simulink model "PubIfDecisionTOS_MDL"  (R2020b)
settings: configuration reference "DspaceConfig" (kept outside this file)
PostLoadFcn:
  | if any(exist('dsrtsu_mdlpostloadfcn', 'file') ~= 0), dsrtsu_mdlpostloadfcn('Execute', bdroot); end
InitFcn:
  | , if any(exist('dsmpb_private', 'file') ~= 0), dsmpb_private('dsmpb_mdlclblib', 'Init', bdroot); end,
undefined symbols (not defined in the file or in its folder): C_TOS_ACCEgoRAxletoFbumplength_m, C_TOS_ACCTargetFront_Flag, C_TOS_AEBJAPedObjDxThre_Val, C_TOS_AEBJAPedObjDyThre_Val, C_TOS_AEBJATargetSize_Val, C_TOS_AEBJAVehObjDxThre_Val, C_TOS_AEBJAVehObjDyThre_Val, C_TOS_AEBJuncPedTargetSize_Val, C_TOS_AEBLatObjDxThre_Val, C_TOS_AEBLatPedDyThre_Val, C_TOS_AEBLatTargetSize_Val, C_TOS_AEBLongTargetInEgoFront_Flag, C_TOS_axAbsGround_Parameter, C_TOS_CameraConfirmedFlag, C_TOS_CNsubjWidth, C_TOS_CurrentLaneCoreMinWidth_Val, C_TOS_CutInProb_Val_Zero, C_TOS_CutOutProb_Val_Zero, C_TOS_D2R_Val, C_TOS_DefaultValueObjectToCenterLine_dy, C_TOS_EgoCarWidth_Val, C_TOS_EgoDxRefPoint_m, C_TOS_EgoRAxletoFbumplength_m, C_TOS_HalfWidthVehicle_Con, C_TOS_HWA_CurrentLaneFlag, C_TOS_HWA_LeftLaneFlag, C_TOS_HWA_MovingDir_Vaild, C_TOS_HWA_MovState_Vaild, C_TOS_HWA_RightLaneFlag, C_TOS_LaneLineCourseErrorFront, C_TOS_LaneLineCourseErrorRear, C_TOS_MotorbikeDefaultWidth_m, C_TOS_NumberOfEffectiveTargets, C_TOS_Obj_Age_Val, C_TOS_Objdx_Constraint_Val, C_TOS_ObjectDefaultWidth_m, C_TOS_ObjInCurrentLane_Val, C_TOS_ObjInCurrentLaneValid, C_TOS_ObjInLeftLaneValid, C_TOS_ObjInRightLaneValid, C_TOS_ObjNotInCurrentLane_Val, C_TOS_ObjNotREElementType, C_TOS_ObjPredictDis_dy_ConstantVal_Zeros, C_TOS_ObjToCenterLine_ConstantVal_Zeros, C_TOS_OFMObjIDInvilad_Val, C_TOS_PIL_LatDisCons_Val_zero, C_TOS_PIL_ObjectCutInFlag_b, C_TOS_PIL_ObjectCutOutFlag_b, C_TOS_PIL_ObjLaneProb_al_Val, C_TOS_PP_ObjFusType_FC_Confirm_b, C_TOS_PP_ObjFusType_FC_FR_Confirm_b, C_TOS_PP_ObjFusType_FR_Confirm_b, C_TOS_RE_80BoolDefault_Val, C_TOS_RE_80Single181Default_Val, C_TOS_RE_80Single255Default_Val, C_TOS_RE_80Uint8Default_Val, C_TOS_RE_D2R, C_TOS_RE_D_180_Val, C_TOS_RE_InvalidObjectID_Val, C_TOS_RE_InvalidTargetChainDir_Val ... (+142)
libraries: simulink x1650, TOS_LIB x361, canfdmsglib x14
(part 14 of 69)

== system PubIfDecisionTOS_MDL/TOS_20201112/TOS_2012080320/TOS/P0_Trajectory_V1.0/CordinatConvert/CordinatConvert1 ==
  note: 0x0: not standstill
  EgoVeh_OffsetX : Inport
  EgoVeh_OffsetY : Inport  Port=2
  EgoVeh_OffsetAngle : Inport  Port=3
  VxvRef_ms : Inport  Port=4
  VehStandstill : Inport  Port=5
  P0_dx_TrackRecord_K1 : Inport  Port=6
  P0_dy_TrackRecord_K1 : Inport  Port=7
  P0_Counter_TrackRecord_K1 : Inport  Port=8
  P0_ID_TrackRecord_K1 : Inport  Port=9
  Bus Creator : BusCreator  Inputs=9
  Bus Selector : BusSelector  OutputSignals=VehStandstill
  Bus Selector1 : BusSelector  OutputSignals=EgoVeh_OffsetX,EgoVeh_OffsetY,EgoVeh_OffsetAngle,P0_dx_TrackRecord_K1,P0_dy_TrackRecord_K1,P0_Counter_TrackRecord_K1,P0_ID_TrackRecord_K1
  Bus Selector2 : BusSelector  OutputSignals=VxvRef_ms
  Compare To Constant1 : simulink/Logic and Bit Operations/Compare To Constant  relop===  const=boolean(0)  OutDataTypeStr=boolean
      settings: AttributesFormatString=boolean(0)
  Compare To Constant2 : simulink/Logic and Bit Operations/Compare To Constant  relop=<  const=single(0.4166)  OutDataTypeStr=boolean
      settings: AttributesFormatString=single(0.4166)
  CordinatConvert : Subsystem  TreatAsAtomicUnit=on
  CordinatConvertDefault : Subsystem  TreatAsAtomicUnit=on
  If : If  IfExpression=u1 == 0
  Logical Operator2 : Logic  Operator=OR  AllPortsSameDT=off  OutDataTypeStr=boolean
  Merge{1..4} (4 alike) : Merge
  P0_dx_TrackRecord_CordinatConvert_K1 : Outport
  P0_dy_TrackRecord_CordinatConvert_K1 : Outport  Port=2
  P0_Counter_TrackRecord_CordinatConvert_K1 : Outport  Port=3
  P0_ID_TrackRecord_CordinatConvert_K1 : Outport  Port=4
  wires:
  Compare To Constant1/1 -> Logical Operator2/1
  Logical Operator2/1 -> If/1
  Compare To Constant2/1 -> Logical Operator2/2
  Bus Selector2/1 -> Compare To Constant2/1  "<VxvRef_ms>"
  VxvRef_ms/1 -> Bus Creator/4  "VxvRef_ms"
  CordinatConvert/4(P0_ID_TrackRecord_CordinatConvert_K1) -> Merge4/1
  CordinatConvertDefault/4(P0_ID_TrackRecord_CordinatConvert_K1) -> Merge4/2
  Merge4/1 -> P0_ID_TrackRecord_CordinatConvert_K1/1
  Bus Selector1/7 -> CordinatConvert/7(P0_ID_TrackRecord_K1)  "<P0_ID_TrackRecord_K1>"
  P0_ID_TrackRecord_K1/1 -> Bus Creator/9  "P0_ID_TrackRecord_K1"
  If/2 -> CordinatConvertDefault/Action
  If/1 -> CordinatConvert/Action
  EgoVeh_OffsetX/1 -> Bus Creator/1  "EgoVeh_OffsetX"
  EgoVeh_OffsetY/1 -> Bus Creator/2  "EgoVeh_OffsetY"
  EgoVeh_OffsetAngle/1 -> Bus Creator/3  "EgoVeh_OffsetAngle"
  VehStandstill/1 -> Bus Creator/5  "VehStandstill"
  P0_dx_TrackRecord_K1/1 -> Bus Creator/6  "P0_dx_TrackRecord_K1"
  P0_dy_TrackRecord_K1/1 -> Bus Creator/7  "P0_dy_TrackRecord_K1"
  P0_Counter_TrackRecord_K1/1 -> Bus Creator/8  "P0_Counter_TrackRecord_K1"
  Bus Creator/1 -> [CordinatConvert_Sig], Bus Selector/1, Bus Selector2/1
  Bus Selector/1 -> Compare To Constant1/1  "<VehStandstill>"
  [CordinatConvert_Sig] -> Bus Selector1/1
  CordinatConvertDefault/3(P0_Counter_TrackRecord_CordinatConvert_K1) -> Merge1/2
  CordinatConvertDefault/2(P0_dy_TrackRecord_CordinatConvert_K1) -> Merge3/2
  CordinatConvertDefault/1(P0_dx_TrackRecord_CordinatConvert_K1) -> Merge2/2
  Bus Selector1/1 -> CordinatConvert/1(EgoVeh_OffsetX)  "<EgoVeh_OffsetX>"
  Bus Selector1/2 -> CordinatConvert/2(EgoVeh_OffsetY)  "<EgoVeh_OffsetY>"
  Bus Selector1/3 -> CordinatConvert/3(EgoVeh_OffsetAngle)  "<EgoVeh_OffsetAngle>"
  Bus Selector1/4 -> CordinatConvert/4(P0_dx_TrackRecord_K1)  "<P0_dx_TrackRecord_K1>"
  Bus Selector1/5 -> CordinatConvert/5(P0_dy_TrackRecord_K1)  "<P0_dy_TrackRecord_K1>"
  Bus Selector1/6 -> CordinatConvert/6(P0_Counter_TrackRecord)  "<P0_Counter_TrackRecord_K1>"
  CordinatConvert/1(P0_dx_TrackRecord_CordinatConvert_K1) -> Merge2/1
  CordinatConvert/2(P0_dy_TrackRecord_CordinatConvert_K1) -> Merge3/1
  CordinatConvert/3(P0_Counter_TrackRecord_CordinatConvert_K1) -> Merge1/1
  Merge2/1 -> P0_dx_TrackRecord_CordinatConvert_K1/1
  Merge3/1 -> P0_dy_TrackRecord_CordinatConvert_K1/1
  Merge1/1 -> P0_Counter_TrackRecord_CordinatConvert_K1/1

== system PubIfDecisionTOS_MDL/TOS_20201112/TOS_2012080320/TOS/P0_Trajectory_V1.0/CordinatConvert/EgoVehicleOffset ==
  note: rcs-reference coordinate system
  PsiDtOpt : Inport
  VxvRef_ms : Inport  Port=2
  Compare To Zero : simulink/Logic and Bit Operations/Compare To Zero  relop===  OutDataTypeStr=boolean
  Constant3 : Constant  Value=0  OutDataTypeStr=single
  Constant4 : Constant  Value=P_TOS_SysCycTime_Val
  Constant5 : Constant  OutDataTypeStr=single
  Constant6 : Constant  Value=P_TOS_SysCycTime_Val
  Constant7 : Constant  Value=0  OutDataTypeStr=boolean
  Constant8 : Constant  Value=0.0000000001  OutDataTypeStr=single
  Divide : Product  Inputs=*/
  DocBlock : simulink/Model-Wide Utilities/DocBlock  DocumentType=Text
      content=|
      | ## author:
      | livie
      | ## Data:
      | Nov 5,2019
      | ## Description:
      | calculate the offset of vehicle coordinate system in x、y、z direction
  Math Function1 : Math  Operator=square  SignedPower=on  SaturateOnIntegerOverflow=on
  Product{,1..4} (5 alike) : Product
  Subtract : Sum  Inputs=+-
  Switch1 : Switch  Criteria=u2 ~= 0
  Switch2 : Switch  Criteria=u2 ~= 0
  Switch3 : Switch  Criteria=u2 ~= 0
  Switch4 : Switch  Criteria=u2 > Threshold
  Trigonometric Function : Trigonometry  Operator=cos
  Trigonometric Function1 : Trigonometry
  EgoVeh_OffsetX : Outport
  EgoVeh_OffsetY : Outport  Port=2
  EgoVeh_OffsetAngle : Outport  Port=3
  wires:
  Switch4/1 -> Product1/1, Product/2
  VxvRef_ms/1 -> Product/1, Math Function1/1, Product3/1
  Math Function1/1 -> Divide/1
  Product/1 -> Divide/2  "ay"
  Constant7/1 -> Switch3/2, Switch2/2, Switch1/2
  Switch1/1 -> EgoVeh_OffsetAngle/1  "rcsoffsetAng"
  Constant3/1 -> Switch1/1, Switch2/1
  Constant4/1 -> Product1/2
  Product1/1 -> Trigonometric Function1/1, Trigonometric Function/1, Switch1/3
  Switch2/1 -> EgoVeh_OffsetY/1
  Switch3/1 -> EgoVeh_OffsetX/1
  Divide/1 -> Product4/1, Product2/1  "R"
  Subtract/1 -> Product2/2
  Constant5/1 -> Subtract/1
  Trigonometric Function/1 -> Subtract/2
  Product2/1 -> Switch2/3
  Constant6/1 -> Product3/2
  Product3/1 -> Switch3/1
  Trigonometric Function1/1 -> Product4/2
  Product4/1 -> Switch3/3
  PsiDtOpt/1 -> Switch4/3, Compare To Zero/1
  Compare To Zero/1 -> Switch4/2
  Constant8/1 -> Switch4/1

== system PubIfDecisionTOS_MDL/TOS_20201112/TOS_2012080320/TOS/P0_Trajectory_V1.0/DataConfirm/Subsystem2 ==
  P0_dx_TrackRecord : Inport
  P0_dy_TrackRecord : Inport  Port=2
  P0_Counter_TrackRecord : Inport  Port=3
  P0_StartPosition_Num : Inport  Port=4
  P0_EndPosition_Num : Inport  Port=5
  Action Port : ActionPort  ActionPortLabel=if(u1 == 1)
  For Iterator Subsystem : Subsystem  TreatAsAtomicUnit=on
  dx : Outport
  dy : Outport  Port=2
  P0_Counter : Outport  Port=3
  wires:
  For Iterator Subsystem/1(dx) -> dx/1
  For Iterator Subsystem/2(dy) -> dy/1
  For Iterator Subsystem/3(P0_Counter) -> P0_Counter/1
  P0_StartPosition_Num/1 -> For Iterator Subsystem/4(P0_StartPosition_Num)
  P0_dx_TrackRecord/1 -> For Iterator Subsystem/1(P0_dx_TrackRecord)
  P0_dy_TrackRecord/1 -> For Iterator Subsystem/2(P0_dy_TrackRecord)
  P0_Counter_TrackRecord/1 -> For Iterator Subsystem/3(P0_Counter_TrackRecord)
  P0_EndPosition_Num/1 -> For Iterator Subsystem/5(P0_EndPosition_Num)

== system PubIfDecisionTOS_MDL/TOS_20201112/TOS_2012080320/TOS/P0_Trajectory_V1.0/DataConfirm/Subsystem3 ==
  P0_dx_TrackRecord : Inport
  P0_dy_TrackRecord : Inport  Port=2
  P0_Counter_TrackRecord : Inport  Port=3
  P0_StartPosition_Num : Inport  Port=4
  P0_EndPosition_Num : Inport  Port=5
  Action Port : ActionPort  ActionPortLabel=else
  For Iterator Subsystem : Subsystem  TreatAsAtomicUnit=on
  dx : Outport
  dy : Outport  Port=2
  P0_Counter : Outport  Port=3
  wires:
  P0_EndPosition_Num/1 -> For Iterator Subsystem/5(P0_EndPosition_Num)
  P0_Counter_TrackRecord/1 -> For Iterator Subsystem/3(P0_Counter_TrackRecord)
  P0_dy_TrackRecord/1 -> For Iterator Subsystem/2(P0_dy_TrackRecord)
  P0_dx_TrackRecord/1 -> For Iterator Subsystem/1(P0_dx_TrackRecord)
  P0_StartPosition_Num/1 -> For Iterator Subsystem/4(P0_StartPosition_Num)
  For Iterator Subsystem/3(P0_Counter) -> P0_Counter/1
  For Iterator Subsystem/2(dy) -> dy/1
  For Iterator Subsystem/1(dx) -> dx/1

== system PubIfDecisionTOS_MDL/TOS_20201112/TOS_2012080320/TOS/P0_Trajectory_V1.0/TrackRecord/Subsystem1 ==
  note: 未填满80位时，一定存在0值；
  note: 存在0值
  TrackRecord_Sig : Inport
  Action Port : ActionPort  ActionPortLabel=else
  Bus Creator : BusCreator  Inputs=5
  Bus Creator1 : BusCreator  Inputs=5
  Bus Selector : BusSelector  OutputSignals=P0_StartPosition_Num,P0_StartPosition_Dis,P0_EndPosition_Num,P0_EndPosition_dx,P0_EndPosition_dy
  Bus Selector1 : BusSelector  OutputSignals=TrackRecord_CordinatConvert.P0_dx_TrackRecord_CordinatConvert_K1
  Bus Selector2 : BusSelector  OutputSignals=TrackRecord_CordinatConvert.P0_dy_TrackRecord_CordinatConvert_K1
  Bus Selector3 : BusSelector  OutputSignals=TrackRecord_CordinatConvert.P0_ID_TrackRecord_CordinatConvert_K1
  Bus Selector4 : BusSelector  OutputSignals=TrackRecord_CordinatConvert.P0_Counter_TrackRecord_CordinatConvert_K1
  Bus Selector7 : BusSelector  OutputSignals=TrackRecord_CordinatConvert.P0_dx_TrackRecord_CordinatConvert_K1,TrackRecord_CordinatConvert.P0_dy_TrackRecord_CordinatConvert_K1,TrackRecord_CordinatConvert.P0_Counter_TrackRecord_CordinatConvert_K1
  Bus Selector8 : BusSelector  OutputSignals=TrackRecord_CordinatConvert.P0_dx_TrackRecord_CordinatConvert_K1,TrackRecord_CordinatConvert.P0_dy_TrackRecord_CordinatConvert_K1,TrackRecord_CordinatConvert.P0_Counter_TrackRecord_CordinatConvert_K1
  Constant6 : Constant  Value=P_TOS_P0_Trajectory_TrackRecord_Num  OutDataTypeStr=uint32
      settings: AttributesFormatString=P0_Trajectory_TrackRecord_Num = unit32(60)
  MATLAB Function : MATLAB Function  TreatAsAtomicUnit=on
  MATLAB Function1 : MATLAB Function  TreatAsAtomicUnit=on
  P0_Position_Num : Subsystem
  Signal Copy{,1..3} (4 alike) : SignalConversion  OverrideOpt=off
  Switch : Switch  Criteria=u2 > Threshold
  P0_dx_TrackRecord : Outport
  P0_dy_TrackRecord : Outport  Port=2
  P0_Counter_TrackRecord : Outport  Port=3
  P0_StartPosition_Num : Outport  Port=4
  P0_EndPosition_Num : Outport  Port=5
  P0_ID_TrackRecord : Outport  Port=6
  P0_StartPosition_Dis : Outport  Port=7
  P0_EndPosition_dx : Outport  Port=8
  P0_EndPosition_dy : Outport  Port=9
  wires:
  Bus Selector4/1 -> Signal Copy2/1  "<P0_Counter_TrackRecord_CordinatConvert_K1>"
  Bus Selector2/1 -> Signal Copy1/1  "<P0_dy_TrackRecord_CordinatConvert_K1>"
  Bus Selector1/1 -> Signal Copy/1  "<P0_dx_TrackRecord_CordinatConvert_K1>"
  Signal Copy/1 -> P0_dx_TrackRecord/1  "P0_dx_TrackRecord"
  Signal Copy1/1 -> P0_dy_TrackRecord/1  "P0_dy_TrackRecord"
  Signal Copy2/1 -> P0_Counter_TrackRecord/1  "P0_Counter_TrackRecord"
  Bus Selector3/1 -> Signal Copy3/1  "<P0_ID_TrackRecord_CordinatConvert_K1>"
  Signal Copy3/1 -> P0_ID_TrackRecord/1
  P0_Position_Num/2(P0_StartPosition_Dis) -> Bus Creator/2  "P0_StartPosition_Dis"
  MATLAB Function/1(EmptyDataConfirm) -> Switch/2
  Bus Creator/1 -> Switch/1
  Bus Selector7/2 -> MATLAB Function/2(P0_dy_TrackRecord_CordinatConvert_K1), P0_Position_Num/2(P0_dy_TrackRecord_CordinatConvert_K1)  "<P0_dy_TrackRecord_CordinatConvert_K1>"
  Switch/1 -> Bus Selector/1
  Bus Selector7/1 -> MATLAB Function/1(P0_dx_TrackRecord_CordinatConvert_K1), P0_Position_Num/1(P0_dx_TrackRecord_CordinatConvert_K1)  "<P0_dx_TrackRecord_CordinatConvert_K1>"
  P0_Position_Num/1(P0_StartPosition_Num) -> Bus Creator/1  "P0_StartPosition_Num"
  TrackRecord_Sig/1 -> Bus Selector7/1, Bus Selector8/1, Bus Selector4/1, Bus Selector2/1, Bus Selector1/1, Bus Selector3/1
  Constant6/1 -> MATLAB Function/4(P0_Trajectory_TrackRecord_Num), P0_Position_Num/4(P0_Trajectory_TrackRecord_Num)
  Bus Creator1/1 -> Switch/3
  Bus Selector7/3 -> MATLAB Function/3(P0_Counter_TrackRecord_CordinatConvert_K1), P0_Position_Num/3(P0_ObjVaild_TrackRecord_CordinatConvert_K1)  "<P0_Counter_TrackRecord_CordinatConvert_K1>"
  P0_Position_Num/3(P0_EndPosition_Num) -> Bus Creator/3  "P0_EndPosition_Num"
  P0_Position_Num/4(P0_EndPosition_dx) -> Bus Creator/4  "P0_EndPosition_dx"
  P0_Position_Num/5(P0_EndPosition_dy) -> Bus Creator/5  "P0_EndPosition_dy"
  MATLAB Function1/3(P0_EndPosition_Num) -> Bus Creator1/3  "P0_EndPosition_Num"
  MATLAB Function1/1(P0_StartPosition_Num) -> Bus Creator1/1  "P0_StartPosition_Num"
  MATLAB Function1/2(P0_StartPosition_Dis) -> Bus Creator1/2  "P0_StartPosition_Dis"
  MATLAB Function1/4(P0_EndPosition_dx) -> Bus Creator1/4  "P0_EndPosition_dx"
  MATLAB Function1/5(P0_EndPosition_dy) -> Bus Creator1/5  "P0_EndPosition_dy"
  Bus Selector/1 -> P0_StartPosition_Num/1  "<P0_StartPosition_Num>"
  Bus Selector/2 -> P0_StartPosition_Dis/1  "<P0_StartPosition_Dis>"
  Bus Selector/3 -> P0_EndPosition_Num/1  "<P0_EndPosition_Num>"
  Bus Selector/4 -> P0_EndPosition_dx/1  "<P0_EndPosition_dx>"
  Bus Selector/5 -> P0_EndPosition_dy/1  "<P0_EndPosition_dy>"
  Bus Selector8/2 -> MATLAB Function1/2(P0_dy_TrackRecord_CordinatConvert_K1)  "<P0_dy_TrackRecord_CordinatConvert_K1>"
  Bus Selector8/1 -> MATLAB Function1/1(P0_dx_TrackRecord_CordinatConvert_K1)  "<P0_dx_TrackRecord_CordinatConvert_K1>"
  Bus Selector8/3 -> MATLAB Function1/3(P0_Counter_TrackRecord_CordinatConvert_K1)  "<P0_Counter_TrackRecord_CordinatConvert_K1>"

== system PubIfDecisionTOS_MDL/TOS_20201112/TOS_2012080320/TOS/P0_Trajectory_V1.0/TrackRecord/Subsystem2 ==
  P0_Index : Inport
  TrackRecord_Sig : Inport  Port=2
  Action Port : ActionPort  ActionPortLabel=if(u1 == 1)
  Assignment{1..4} (4 alike) : Assignment  DiagnosticForDimensions=Warning  IndexOptions=Index vector (port)  Indices=1  OutputSizes=1
  Bus Creator : BusCreator  Inputs=2
  Bus Creator1 : BusCreator  Inputs=2
  Bus Selector : BusSelector  OutputSignals=P0_StartPosition_Num,P0_StartPosition_Dis
  Bus Selector1 : BusSelector  OutputSignals=TrackRecord_CordinatConvert.P0_dx_TrackRecord_CordinatConvert_K1,TOS_ACC_P0_Inf.P0_dx
  Bus Selector2 : BusSelector  OutputSignals=TrackRecord_CordinatConvert.P0_dy_TrackRecord_CordinatConvert_K1,TOS_ACC_P0_Inf.P0_dy
  Bus Selector3 : BusSelector  OutputSignals=TrackRecord_CordinatConvert.P0_ID_TrackRecord_CordinatConvert_K1,TOS_ACC_P0_Inf.P0_ID
  Bus Selector4 : BusSelector  OutputSignals=TrackRecord_CordinatConvert.P0_Counter_TrackRecord_CordinatConvert_K1,TOS_ACC_P0_Inf.P0_Counter
  Bus Selector5 : BusSelector  OutputSignals=TOS_ACC_P0_Inf.P0_dx,TOS_ACC_P0_Inf.P0_dy
  Bus Selector6 : BusSelector  OutputSignals=TrackRecord_CordinatConvert.P0_dx_TrackRecord_CordinatConvert_K1
  Bus Selector7 : BusSelector  OutputSignals=TrackRecord_CordinatConvert.P0_dx_TrackRecord_CordinatConvert_K1,TrackRecord_CordinatConvert.P0_dy_TrackRecord_CordinatConvert_K1,TrackRecord_CordinatConvert.P0_Counter_TrackRecord_CordinatConvert_K1
  Constant{1..4} (4 alike) : Constant  Value=P_TOS_P0_Trajectory_TrackRecord_Num  OutDataTypeStr=uint32
      settings: AttributesFormatString=P0_Trajectory_TrackRecord_Num = unit32(60)
  MATLAB Function : MATLAB Function  TreatAsAtomicUnit=on
  P0_Position_Num : Subsystem
  Selector : Selector  InputPortWidth=80  IndexOptions=Index vector (port)  Indices=[1 3]  OutputSizes=1
  Switch : Switch  Criteria=u2 > Threshold
  P0_dx_TrackRecord : Outport
  P0_dy_TrackRecord : Outport  Port=2
  P0_Counter_TrackRecord : Outport  Port=3
  P0_StartPosition_Num : Outport  Port=4
  P0_EndPosition_Num : Outport  Port=5
  P0_ID_TrackRecord : Outport  Port=6
  P0_StartPosition_Dis : Outport  Port=7
  P0_EndPosition_dx : Outport  Port=8
  P0_EndPosition_dy : Outport  Port=9
  wires:
  Constant1/1 -> P0_EndPosition_Num/1  "P0_EndPosition_Num"
  P0_Position_Num/1(P0_StartPosition_Num) -> Bus Creator/1  "P0_StartPosition_Num"
  Bus Selector4/2 -> Assignment3/2  "<P0_Counter>"
  Bus Selector1/1 -> Assignment1/1  "<P0_dx_TrackRecord_CordinatConvert_K1>"
  Bus Selector4/1 -> Assignment3/1  "<P0_Counter_TrackRecord_CordinatConvert_K1>"
  Bus Selector1/2 -> Assignment1/2  "<P0_dx>"
  P0_Index/1 -> Assignment4/3, Assignment3/3, Assignment2/3, Assignment1/3
  Bus Selector2/2 -> Assignment2/2  "<P0_dy>"
  Bus Selector2/1 -> Assignment2/1  "<P0_dy_TrackRecord_CordinatConvert_K1>"
  Assignment1/1 -> P0_dx_TrackRecord/1  "P0_dx_TrackRecord"
  Assignment2/1 -> P0_dy_TrackRecord/1  "P0_dy_TrackRecord"
  Assignment3/1 -> P0_Counter_TrackRecord/1  "P0_Counter_TrackRecord"
  Assignment4/1 -> P0_ID_TrackRecord/1
  Bus Selector3/2 -> Assignment4/2  "<P0_ID>"
  Bus Selector3/1 -> Assignment4/1  "<P0_ID_TrackRecord_CordinatConvert_K1>"
  Bus Selector7/2 -> MATLAB Function/2(P0_dy_TrackRecord_CordinatConvert_K1), P0_Position_Num/2(P0_dy_TrackRecord_CordinatConvert_K1)  "<P0_dy_TrackRecord_CordinatConvert_K1>"
  Bus Selector7/3 -> MATLAB Function/3(P0_Counter_TrackRecord_CordinatConvert_K1), P0_Position_Num/3(P0_ObjVaild_TrackRecord_CordinatConvert_K1)  "<P0_Counter_TrackRecord_CordinatConvert_K1>"
  Bus Selector7/1 -> MATLAB Function/1(P0_dx_TrackRecord_CordinatConvert_K1), P0_Position_Num/1(P0_dx_TrackRecord_CordinatConvert_K1)  "<P0_dx_TrackRecord_CordinatConvert_K1>"
  Constant2/1 -> MATLAB Function/4(P0_Trajectory_TrackRecord_Num), P0_Position_Num/4(P0_Trajectory_TrackRecord_Num)
  Bus Selector5/1 -> P0_EndPosition_dx/1  "<P0_dx>"
  TrackRecord_Sig/1 -> [TrackRecord_Sig], Bus Selector5/1, Bus Selector7/1, Bus Selector3/1, Bus Selector4/1, Bus Selector2/1, Bus Selector1/1
  P0_Position_Num/2(P0_StartPosition_Dis) -> Bus Creator/2  "P0_StartPosition_Dis"
  Bus Selector5/2 -> P0_EndPosition_dy/1  "<P0_dy>"
  Switch/1 -> Bus Selector/1
  Bus Creator/1 -> Switch/1
  MATLAB Function/1(EmptyDataConfirm) -> Switch/2
  Bus Creator1/1 -> Switch/3
  Selector/1 -> Bus Creator1/2  "P0_StartPosition_Dis"
  Constant3/1 -> Bus Creator1/1  "P0_StartPosition_Num"
  Bus Selector/2 -> P0_StartPosition_Dis/1  "<P0_StartPosition_Dis>"
  Bus Selector/1 -> P0_StartPosition_Num/1  "<P0_StartPosition_Num>"
  Constant4/1 -> Selector/2
  [TrackRecord_Sig] -> Bus Selector6/1
  Bus Selector6/1 -> Selector/1  "<P0_dx_TrackRecord_CordinatConvert_K1>"

== system PubIfDecisionTOS_MDL/TOS_20201112/TOS_2012080320/TOS/P0_Trajectory_V1.0/TrackRecord/Subsystem3 ==
  note: 未填满80位时，一定存在0值；
  note: 存在0值
  P0_Index : Inport
  TrackRecord_Sig : Inport  Port=2
  Action Port : ActionPort  ActionPortLabel=elseif(u2 == 1)
  Add2 : Sum
  Assignment{1..4} (4 alike) : Assignment  DiagnosticForDimensions=Warning  IndexOptions=Index vector (port)  Indices=1  OutputSizes=1
  Bus Creator : BusCreator  Inputs=2
  Bus Creator3 : BusCreator  Inputs=2
  Bus Selector : BusSelector  OutputSignals=P0_StartPosition_Num,P0_StartPosition_Dis
  Bus Selector1 : BusSelector  OutputSignals=TrackRecord_CordinatConvert.P0_dx_TrackRecord_CordinatConvert_K1,TOS_ACC_P0_Inf.P0_dx
  Bus Selector2 : BusSelector  OutputSignals=TrackRecord_CordinatConvert.P0_dy_TrackRecord_CordinatConvert_K1,TOS_ACC_P0_Inf.P0_dy
  Bus Selector3 : BusSelector  OutputSignals=TOS_ACC_P0_Inf.P0_dx,TOS_ACC_P0_Inf.P0_dy
  Bus Selector4 : BusSelector  OutputSignals=TrackRecord_CordinatConvert.P0_Counter_TrackRecord_CordinatConvert_K1,TOS_ACC_P0_Inf.P0_Counter
  Bus Selector6 : BusSelector  OutputSignals=TrackRecord_CordinatConvert.P0_ID_TrackRecord_CordinatConvert_K1,TOS_ACC_P0_Inf.P0_ID
  Bus Selector7 : BusSelector  OutputSignals=TrackRecord_CordinatConvert.P0_dx_TrackRecord_CordinatConvert_K1,TrackRecord_CordinatConvert.P0_dy_TrackRecord_CordinatConvert_K1,TrackRecord_CordinatConvert.P0_Counter_TrackRecord_CordinatConvert_K1
  Bus Selector8 : BusSelector  OutputSignals=TrackRecord_CordinatConvert.P0_dx_TrackRecord_CordinatConvert_K1
  Constant2 : Constant  Value=P_TOS_P0_Trajectory_TrackRecord_Num  OutDataTypeStr=uint32
      settings: AttributesFormatString=P0_Trajectory_TrackRecord_Num = unit32(60)
  Constant3 : Constant  Value=uint32(1)  OutDataTypeStr=uint32
      settings: AttributesFormatString=uint32(1)
  MATLAB Function : MATLAB Function  TreatAsAtomicUnit=on
  P0_Position_Num : Subsystem
  Selector1 : Selector  InputPortWidth=80  IndexOptions=Index vector (port)  Indices=[1 3]  OutputSizes=1
  Switch : Switch  Criteria=u2 > Threshold
  P0_dx_TrackRecord : Outport
  P0_dy_TrackRecord : Outport  Port=2
  P0_Counter_TrackRecord : Outport  Port=3
  P0_StartPosition_Num : Outport  Port=4
  P0_EndPosition_Num : Outport  Port=5
  P0_ID_TrackRecord : Outport  Port=6
  P0_StartPosition_Dis : Outport  Port=7
  P0_EndPosition_dx : Outport  Port=8
  P0_EndPosition_dy : Outport  Port=9
  wires:
  Bus Selector6/1 -> Assignment4/1  "<P0_ID_TrackRecord_CordinatConvert_K1>"
  P0_Index/1 -> [P0_Index_Sig], Assignment3/3, Assignment4/3, Assignment2/3, Assignment1/3
  Bus Selector6/2 -> Assignment4/2  "<P0_ID>"
  Assignment4/1 -> P0_ID_TrackRecord/1
  Bus Selector4/2 -> Assignment3/2  "<P0_Counter>"
  Bus Selector1/1 -> Assignment1/1  "<P0_dx_TrackRecord_CordinatConvert_K1>"
  Bus Selector4/1 -> Assignment3/1  "<P0_Counter_TrackRecord_CordinatConvert_K1>"
  Bus Selector1/2 -> Assignment1/2  "<P0_dx>"
  Bus Selector2/2 -> Assignment2/2  "<P0_dy>"
  Bus Selector2/1 -> Assignment2/1  "<P0_dy_TrackRecord_CordinatConvert_K1>"
  Assignment1/1 -> P0_dx_TrackRecord/1  "P0_dx_TrackRecord"
  Assignment2/1 -> P0_dy_TrackRecord/1  "P0_dy_TrackRecord"
  Assignment3/1 -> P0_Counter_TrackRecord/1  "P0_Counter_TrackRecord"
  [P0_Index_Sig] -> P0_EndPosition_Num/1  "P0_EndPosition_Num"
  Bus Selector3/1 -> P0_EndPosition_dx/1  "<P0_dx>"
  Bus Selector3/2 -> P0_EndPosition_dy/1  "<P0_dy>"
  Bus Selector/2 -> P0_StartPosition_Dis/1  "<P0_StartPosition_Dis>"
  Bus Creator3/1 -> Switch/3
  Bus Selector7/2 -> MATLAB Function/2(P0_dy_TrackRecord_CordinatConvert_K1), P0_Position_Num/2(P0_dy_TrackRecord_CordinatConvert_K1)  "<P0_dy_TrackRecord_CordinatConvert_K1>"
  MATLAB Function/1(EmptyDataConfirm) -> Switch/2
  Bus Selector7/1 -> MATLAB Function/1(P0_dx_TrackRecord_CordinatConvert_K1), P0_Position_Num/1(P0_dx_TrackRecord_CordinatConvert_K1)  "<P0_dx_TrackRecord_CordinatConvert_K1>"
  Bus Selector7/3 -> MATLAB Function/3(P0_Counter_TrackRecord_CordinatConvert_K1), P0_Position_Num/3(P0_ObjVaild_TrackRecord_CordinatConvert_K1)  "<P0_Counter_TrackRecord_CordinatConvert_K1>"
  Bus Creator/1 -> Switch/1
  Constant2/1 -> MATLAB Function/4(P0_Trajectory_TrackRecord_Num), P0_Position_Num/4(P0_Trajectory_TrackRecord_Num)
  Switch/1 -> Bus Selector/1
  Bus Selector/1 -> P0_StartPosition_Num/1  "<P0_StartPosition_Num>"
  P0_Position_Num/2(P0_StartPosition_Dis) -> Bus Creator/2  "P0_StartPosition_Dis"
  P0_Position_Num/1(P0_StartPosition_Num) -> Bus Creator/1  "P0_StartPosition_Num"
  TrackRecord_Sig/1 -> Bus Selector4/1, Bus Selector8/1, Bus Selector7/1, Bus Selector3/1, Bus Selector6/1, Bus Selector2/1, Bus Selector1/1
  Add2/1 -> Bus Creator3/1, Selector1/2  "P0_StartPosition_Num"
  Selector1/1 -> Bus Creator3/2  "P0_StartPosition_Dis"
  Bus Selector8/1 -> Selector1/1  "<P0_dx_TrackRecord_CordinatConvert_K1>"
  [P0_Index_Sig] -> Add2/2  "P0_EndPosition_Num"
  Constant3/1 -> Add2/1

== system PubIfDecisionTOS_MDL/TOS_20201112/TOS_2012080320/TOS/P0_Trajectory_V1.0/TrgValidConfirm/TrgValidConfirm ==
  note: 目标是否有效
  P0_ID_K1 : Inport
  P0_Counter_K1 : Inport  Port=2
  P0_dx_K1 : Inport  Port=3
  TOS_ACC_P0 : Inport  Port=4
  Bus Creator : BusCreator  Inputs=4
  Bus Selector : BusSelector  OutputSignals=TOS_ACC_P0.IDP0,TOS_ACC_P0.ObjMovingStateP0,TOS_ACC_P0.dxP0
  Bus Selector1 : BusSelector  OutputSignals=TOS_ACC_P0.dxP0,TOS_ACC_P0.ObjDYP0,TOS_ACC_P0.IDP0,P0_ID_K1,P0_Counter_K1,P0_dx_K1
  Compare To Constant : simulink/Logic and Bit Operations/Compare To Constant  relop=~=  const=C_TOS_OFMObjIDInvilad_Val  OutDataTypeStr=boolean
      settings: AttributesFormatString=C_TOS_OFMObjIDInvilad_Val = 0
  Compare To Constant2 : simulink/Logic and Bit Operations/Compare To Constant  relop=<=  const=single(80)  OutDataTypeStr=boolean
      settings: AttributesFormatString=single(80)
  Compare To Constant5 : simulink/Logic and Bit Operations/Compare To Constant  relop===  const=ObjectMovingState_E.Moving  OutDataTypeStr=boolean
      settings: AttributesFormatString=ObjectMovingState_E.Moving = 2
  Data Type Conversion : DataTypeConversion  OutDataTypeStr=Enum: ObjectMovingState_E
  If : If  IfExpression=u1 == 0
  Logical Operator1 : Logic  Inputs=3  AllPortsSameDT=off  OutDataTypeStr=boolean
  Merge{,1..3} (4 alike) : Merge
  TrgValidConfirm : Subsystem  TreatAsAtomicUnit=on
  TrgValidConfirmDefault : Subsystem  TreatAsAtomicUnit=on
  P0_ID : Outport
  P0_Counter : Outport  Port=2
  P0_dx : Outport  Port=3
  P0_dy : Outport  Port=4
  wires:
  Bus Selector1/6 -> TrgValidConfirm/6(P0_dx_K1)  "<P0_dx_K1>"
  P0_dx_K1/1 -> Bus Creator/3  "P0_dx_K1"
  Bus Selector1/4 -> TrgValidConfirm/4(P0_ID_K1)  "<P0_ID_K1>"
  Bus Selector1/5 -> TrgValidConfirm/5(P0_Counter_K1)  "<P0_Counter_K1>"
  [TrgValidConfirm_Sig] -> Bus Selector1/1
  TOS_ACC_P0/1 -> Bus Creator/4  "TOS_ACC_P0"
  P0_Counter_K1/1 -> Bus Creator/2  "P0_Counter_K1"
  P0_ID_K1/1 -> Bus Creator/1  "P0_ID_K1"
  TrgValidConfirmDefault/4(P0_dy) -> Merge1/1
  TrgValidConfirmDefault/3(P0_dx) -> Merge/1
  TrgValidConfirmDefault/2(P0_Counter) -> Merge2/1
  TrgValidConfirmDefault/1(P0_ID) -> Merge3/1
  Merge3/1 -> P0_ID/1
  TrgValidConfirm/1(P0_ID) -> Merge3/2
  Bus Selector1/3 -> TrgValidConfirm/3(IDP0)  "<IDP0>"
  Data Type Conversion/1 -> Compare To Constant5/1
  Merge2/1 -> P0_Counter/1
  Merge1/1 -> P0_dy/1
  Merge/1 -> P0_dx/1
  TrgValidConfirm/2(P0_Counter) -> Merge2/2
  TrgValidConfirm/4(P0_dy) -> Merge1/2
  TrgValidConfirm/3(P0_dx) -> Merge/2
  Bus Selector1/2 -> TrgValidConfirm/2(ObjDYP0)  "<ObjDYP0>"
  Bus Selector1/1 -> TrgValidConfirm/1(dxP0)  "<dxP0>"
  Logical Operator1/1 -> If/1  "TOS_P0_TARGET_TrgValidConfirm_ObserVale"
  Compare To Constant/1 -> Logical Operator1/1
  If/1 -> TrgValidConfirmDefault/Action
  If/2 -> TrgValidConfirm/Action
  Bus Selector/2 -> Data Type Conversion/1  "<ObjMovingStateP0>"
  Bus Selector/1 -> Compare To Constant/1  "<IDP0>"
  Compare To Constant5/1 -> Logical Operator1/2
  Bus Creator/1 -> [TrgValidConfirm_Sig], Bus Selector/1
  Bus Selector/3 -> Compare To Constant2/1  "<dxP0>"
  Compare To Constant2/1 -> Logical Operator1/3

== system PubIfDecisionTOS_MDL/TOS_20201112/TOS_2012080320/PIL_1029/BoundaryCalculat/Lane_BoundaryCalculat/Lane_Boundary/Boundary ==
  Object_Type : Inport
  Object_DX : Inport  Port=2
  object_MovingState : Inport  Port=3
  PP_CurrentLaneWidth : Inport  Port=4
  PP_LeftLaneWidth : Inport  Port=5
  PP_RightLaneWidth : Inport  Port=6
  C_LaneLineCourseErrorFront : Inport  Port=7
  C_LaneLineCourseErrorRear : Inport  Port=8
  Action Port : ActionPort  ActionPortLabel=else
  Bus Creator : BusCreator  Inputs=8
  Bus Selector : BusSelector  OutputSignals=Object_Type,object_MovingState,PP_CurrentLaneWidth
  Bus Selector1 : BusSelector  OutputSignals=Object_DX,C_LaneLineCourseErrorFront,C_LaneLineCourseErrorRear,PP_CurrentLaneWidth,PP_LeftLaneWidth,PP_RightLaneWidth
  Bus Selector4 : BusSelector  OutputSignals=Object_Type,object_MovingState,PP_LeftLaneWidth
  Bus Selector5 : BusSelector  OutputSignals=Object_Type,object_MovingState,PP_RightLaneWidth
  Bus Selector6 : BusSelector  OutputSignals=Object_DX,C_LaneLineCourseErrorFront,C_LaneLineCourseErrorRear,PP_CurrentLaneWidth,PP_LeftLaneWidth
  Bus Selector7 : BusSelector  OutputSignals=Object_DX,C_LaneLineCourseErrorFront,C_LaneLineCourseErrorRear,PP_CurrentLaneWidth,PP_RightLaneWidth
  LeftLane_BasicLaneWidth : Subsystem
  LeftLane_Boundary : Subsystem
  RightLane_BasicLaneWidth : Subsystem
  RightLane_Boundary : Subsystem
  SameLane_BasicLaneWidth : Subsystem
  SameLane_Boundary : Subsystem
  SameLane_CoreArea_Boundary : Outport
  SameLane_EdgeLeft_Boundary : Outport  Port=2
  SameLane_EdgeRight_Boundary : Outport  Port=3
  LeftLane_CoreArea_Boundary : Outport  Port=4
  LeftLane_EdgeLeft_Boundary : Outport  Port=5
  LeftLane_EdgeRight_Boundary : Outport  Port=6
  RightLane_CoreArea_Boundary : Outport  Port=7
  RightLane_EdgeLeft_Boundary : Outport  Port=8
  RightLane_EdgeRight_Boundary : Outport  Port=9
  SameLane_BasicLaneWidth_ObserVale : Outport  Port=10
  LeftLane_BasicLaneWidth_ObserVale : Outport  Port=11
  RightLane_BasicLaneWidth_ObserVale : Outport  Port=12
  wires:
  [RightLane_BasicLaneWidth] -> RightLane_BasicLaneWidth_ObserVale/1
  [LeftLane_BasicLaneWidth] -> LeftLane_BasicLaneWidth_ObserVale/1
  [SameLane_BasicLaneWidth] -> SameLane_BasicLaneWidth_ObserVale/1
  LeftLane_Boundary/3(LeftLane_EdgeRight_Boundary) -> LeftLane_EdgeRight_Boundary/1
  LeftLane_Boundary/2(LeftLane_EdgeLeft_Boundary) -> LeftLane_EdgeLeft_Boundary/1
  [SameLane_CoreArea_Boundary] -> RightLane_Boundary/6(SameLane_CoreArea_Boundary)
  Bus Selector7/5 -> RightLane_Boundary/5(PP_RightLaneWidth)  "<PP_RightLaneWidth>"
  Bus Selector7/4 -> RightLane_Boundary/4(PP_CurrentLaneWidth)  "<PP_CurrentLaneWidth>"
  Bus Selector6/5 -> LeftLane_Boundary/5(PP_LeftLaneWidth)  "<PP_LeftLaneWidth>"
  Bus Selector6/4 -> LeftLane_Boundary/4(PP_CurrentLaneWidth)  "<PP_CurrentLaneWidth>"
  [RightLane_CoreArea_Boundary] -> SameLane_Boundary/8(RightLane_CoreArea_Boundary)
  [LeftLane_CoreArea_Boundary] -> SameLane_Boundary/7(LeftLane_CoreArea_Boundary)
  Bus Selector1/6 -> SameLane_Boundary/6(PP_RightLaneWidth)  "<PP_RightLaneWidth>"
  Bus Selector1/5 -> SameLane_Boundary/5(PP_LeftLaneWidth)  "<PP_LeftLaneWidth>"
  Bus Selector1/4 -> SameLane_Boundary/4(PP_CurrentLaneWidth)  "<PP_CurrentLaneWidth>"
  RightLane_Boundary/2(RightLane_EdgeLeft_Boundary) -> RightLane_EdgeLeft_Boundary/1
  RightLane_Boundary/3(RightLane_EdgeRight_Boundary) -> RightLane_EdgeRight_Boundary/1
  Bus Creator/1 -> Bus Selector1/1, Bus Selector6/1, Bus Selector7/1, Bus Selector/1, Bus Selector4/1, Bus Selector5/1
  RightLane_Boundary/1(RightLane_CoreArea_Boundary) -> RightLane_CoreArea_Boundary/1, [RightLane_CoreArea_Boundary]
  LeftLane_Boundary/1(LeftLane_CoreArea_Boundary) -> [LeftLane_CoreArea_Boundary], LeftLane_CoreArea_Boundary/1
  [SameLane_CoreArea_Boundary] -> LeftLane_Boundary/6(SameLane_CoreArea_Boundary)
  SameLane_Boundary/3(SameLane_EdgeRight_Boundary) -> SameLane_EdgeRight_Boundary/1
  Bus Selector7/3 -> RightLane_Boundary/3(C_LaneLineCourseErrorRear)  "<C_LaneLineCourseErrorRear>"
  Bus Selector7/1 -> RightLane_Boundary/1(Object_DX)  "<Object_DX>"
  Bus Selector7/2 -> RightLane_Boundary/2(C_LaneLineCourseErrorFront)  "<C_LaneLineCourseErrorFront>"
  RightLane_BasicLaneWidth/1(RightLane_BasicLaneWidth) -> RightLane_Boundary/7(RightLane_BasicLaneWidth), [RightLane_BasicLaneWidth]
  Bus Selector6/3 -> LeftLane_Boundary/3(C_LaneLineCourseErrorRear)  "<C_LaneLineCourseErrorRear>"
  Bus Selector6/2 -> LeftLane_Boundary/2(C_LaneLineCourseErrorFront)  "<C_LaneLineCourseErrorFront>"
  Bus Selector6/1 -> LeftLane_Boundary/1(Object_DX)  "<Object_DX>"
  LeftLane_BasicLaneWidth/1(LeftLane_BasicLaneWidth) -> LeftLane_Boundary/7(LeftLane_BasicLaneWidth), [LeftLane_BasicLaneWidth]
  C_LaneLineCourseErrorFront/1 -> Bus Creator/7
  Bus Selector5/3 -> RightLane_BasicLaneWidth/3(PP_RightLaneWidth)  "<PP_RightLaneWidth>"
  Bus Selector5/2 -> RightLane_BasicLaneWidth/2(object_MovingState)  "<object_MovingState>"
  Bus Selector5/1 -> RightLane_BasicLaneWidth/1(ObjectType)  "<Object_Type>"
  Bus Selector4/3 -> LeftLane_BasicLaneWidth/3(PP_LeftLaneWidth)  "<PP_LeftLaneWidth>"
  Bus Selector4/2 -> LeftLane_BasicLaneWidth/2(object_MovingState)  "<object_MovingState>"
  Bus Selector4/1 -> LeftLane_BasicLaneWidth/1(ObjectType)  "<Object_Type>"
  PP_RightLaneWidth/1 -> Bus Creator/6
  PP_LeftLaneWidth/1 -> Bus Creator/5
  SameLane_Boundary/1(SameLane_CoreArea_Boundary) -> [SameLane_CoreArea_Boundary], SameLane_CoreArea_Boundary/1
  Bus Selector/2 -> SameLane_BasicLaneWidth/2(object_MovingState)  "<object_MovingState>"
  C_LaneLineCourseErrorRear/1 -> Bus Creator/8
  Object_DX/1 -> Bus Creator/2
  PP_CurrentLaneWidth/1 -> Bus Creator/4
  Object_Type/1 -> Bus Creator/1
  Bus Selector1/1 -> SameLane_Boundary/1(Object_DX)  "<Object_DX>"
  object_MovingState/1 -> Bus Creator/3
  Bus Selector/1 -> SameLane_BasicLaneWidth/1(ObjectType)  "<Object_Type>"
  Bus Selector/3 -> SameLane_BasicLaneWidth/3(PP_CurrentLaneWidth)  "<PP_CurrentLaneWidth>"
  SameLane_Boundary/2(SameLane_EdgeLeft_Boundary) -> SameLane_EdgeLeft_Boundary/1
  Bus Selector1/3 -> SameLane_Boundary/3(C_LaneLineCourseErrorRear)  "<C_LaneLineCourseErrorRear>"
  SameLane_BasicLaneWidth/1(BasicLaneWidthOfCurrentLane) -> SameLane_Boundary/9(SameLane_BasicLaneWidth), [SameLane_BasicLaneWidth]
  Bus Selector1/2 -> SameLane_Boundary/2(C_LaneLineCourseErrorFront)  "<C_LaneLineCourseErrorFront>"

== system PubIfDecisionTOS_MDL/TOS_20201112/TOS_2012080320/PIL_1029/BoundaryCalculat/Lane_BoundaryCalculat/Lane_Boundary/BoundaryDefault ==
  Action Port : ActionPort  ActionPortLabel=if(u1 ~= 0)
  Constant{1..12} (12 alike) : Constant  Value=0  OutDataTypeStr=single
  SameLane_CoreArea_Boundary : Outport
  SameLane_EdgeLeft_Boundary : Outport  Port=2
  SameLane_EdgeRight_Boundary : Outport  Port=3
  LeftLane_CoreArea_Boundary : Outport  Port=4
  LeftLane_EdgeLeft_Boundary : Outport  Port=5
  LeftLane_EdgeRight_Boundary : Outport  Port=6
  RightLane_CoreArea_Boundary : Outport  Port=7
  RightLane_EdgeLeft_Boundary : Outport  Port=8
  RightLane_EdgeRight_Boundary : Outport  Port=9
  SameLane_BasicLaneWidth_ObserVale : Outport  Port=10
  LeftLane_BasicLaneWidth_ObserVale : Outport  Port=11
  RightLane_BasicLaneWidth_ObserVale : Outport  Port=12
  wires:
  Constant12/1 -> RightLane_BasicLaneWidth_ObserVale/1
  Constant11/1 -> LeftLane_BasicLaneWidth_ObserVale/1
  Constant10/1 -> SameLane_BasicLaneWidth_ObserVale/1
  Constant9/1 -> RightLane_EdgeRight_Boundary/1
  Constant8/1 -> RightLane_EdgeLeft_Boundary/1
  Constant7/1 -> RightLane_CoreArea_Boundary/1
  Constant6/1 -> LeftLane_EdgeRight_Boundary/1
  Constant5/1 -> LeftLane_EdgeLeft_Boundary/1
  Constant4/1 -> LeftLane_CoreArea_Boundary/1
  Constant3/1 -> SameLane_EdgeRight_Boundary/1
  Constant1/1 -> SameLane_EdgeLeft_Boundary/1
  Constant2/1 -> SameLane_CoreArea_Boundary/1

== system PubIfDecisionTOS_MDL/TOS_20201112/TOS_2012080320/PIL_1029/BoundaryCalculat/ObjectToCenterLine_dyc/LeftLane/LeftCenterLine_dyc ==
  TOS_OFMObjValid_Flag : Inport  Partition=on  PartitionDimension=1  PartitionWidth=1  PartitionOffset=0
  Object_DY : Inport  Port=2  Partition=on  PartitionDimension=1  PartitionWidth=1  PartitionOffset=0
  Object_DX : Inport  Port=3  Partition=on  PartitionDimension=1  PartitionWidth=1  PartitionOffset=0
  line01_C0 : Inport  Port=4
  line01_C1 : Inport  Port=5
  line01_C2 : Inport  Port=6
  line01_C3 : Inport  Port=7
  line01_dDisStart : Inport  Port=8
  line01_dDisEnd : Inport  Port=9
  line02_C0 : Inport  Port=10
  line02_C1 : Inport  Port=11
  line02_C2 : Inport  Port=12
  line02_C3 : Inport  Port=13
  line02_dDisStart : Inport  Port=14
  line02_dDisEnd : Inport  Port=15
  line03_C0 : Inport  Port=16
  line03_C1 : Inport  Port=17
  line03_C2 : Inport  Port=18
  line03_C3 : Inport  Port=19
  line03_dDisStart : Inport  Port=20
  line03_dDisEnd : Inport  Port=21
  line04_C0 : Inport  Port=22
  line04_C1 : Inport  Port=23
  line04_C2 : Inport  Port=24
  line04_C3 : Inport  Port=25
  line04_dDisStart : Inport  Port=26
  line04_dDisEnd : Inport  Port=27
  line05_C0 : Inport  Port=28
  line05_C1 : Inport  Port=29
  line05_C2 : Inport  Port=30
  line05_C3 : Inport  Port=31
  line05_dDisStart : Inport  Port=32
  line05_dDisEnd : Inport  Port=33
  line06_C0 : Inport  Port=34
  line06_C1 : Inport  Port=35
  line06_C2 : Inport  Port=36
  line06_C3 : Inport  Port=37
  line06_dDisStart : Inport  Port=38
  line06_dDisEnd : Inport  Port=39
  Compare To Constant : simulink/Logic and Bit Operations/Compare To Constant  relop===  const=C_TOS_OFMObjIDInvilad_Val  OutDataTypeStr=boolean
      settings: AttributesFormatString=C_TOS_OFMObjIDInvilad_Val = 0
  For Each : ForEach  DisableCoverage=on
  If : If  IfExpression=u1 ~= 0
  Merge : Merge
  ObjToCenterLine_dyc_LeftLane : Subsystem
  ObjToCenterLine_dyc_LeftLaneDefault : Subsystem  TreatAsAtomicUnit=on
  LeftCenterLine_dyc : Outport  ConcatenationDimension=1
  wires:
  ObjToCenterLine_dyc_LeftLaneDefault/1(ObjectToCenterLine_dyc_LeftLane) -> Merge/1
  Merge/1 -> LeftCenterLine_dyc/1
  TOS_OFMObjValid_Flag/1 -> Compare To Constant/1
  If/2 -> ObjToCenterLine_dyc_LeftLane/Action
  Compare To Constant/1 -> If/1
  If/1 -> ObjToCenterLine_dyc_LeftLaneDefault/Action
  ObjToCenterLine_dyc_LeftLane/1(ObjectToCenterLine_dyc_LeftLane) -> Merge/2
  line06_dDisEnd/1 -> ObjToCenterLine_dyc_LeftLane/38(line06_dDisEnd)
  line06_dDisStart/1 -> ObjToCenterLine_dyc_LeftLane/37(line06_dDisStart)
  line06_C3/1 -> ObjToCenterLine_dyc_LeftLane/36(line06_C3)
  line06_C2/1 -> ObjToCenterLine_dyc_LeftLane/35(line06_C2)
  line06_C1/1 -> ObjToCenterLine_dyc_LeftLane/34(line06_C1)
  line06_C0/1 -> ObjToCenterLine_dyc_LeftLane/33(line06_C0)
  line05_dDisEnd/1 -> ObjToCenterLine_dyc_LeftLane/32(line05_dDisEnd)
  line05_dDisStart/1 -> ObjToCenterLine_dyc_LeftLane/31(line05_dDisStart)
  line05_C3/1 -> ObjToCenterLine_dyc_LeftLane/30(line05_C3)
  line05_C2/1 -> ObjToCenterLine_dyc_LeftLane/29(line05_C2)
  line05_C1/1 -> ObjToCenterLine_dyc_LeftLane/28(line05_C1)
  line05_C0/1 -> ObjToCenterLine_dyc_LeftLane/27(line05_C0)
  line04_dDisEnd/1 -> ObjToCenterLine_dyc_LeftLane/26(line04_dDisEnd)
  line04_dDisStart/1 -> ObjToCenterLine_dyc_LeftLane/25(line04_dDisStart)
  line04_C3/1 -> ObjToCenterLine_dyc_LeftLane/24(line04_C3)
  line04_C2/1 -> ObjToCenterLine_dyc_LeftLane/23(line04_C2)
  line04_C1/1 -> ObjToCenterLine_dyc_LeftLane/22(line04_C1)
  line04_C0/1 -> ObjToCenterLine_dyc_LeftLane/21(line04_C0)
  line03_dDisEnd/1 -> ObjToCenterLine_dyc_LeftLane/20(line03_dDisEnd)
  line03_dDisStart/1 -> ObjToCenterLine_dyc_LeftLane/19(line03_dDisStart)
  line03_C3/1 -> ObjToCenterLine_dyc_LeftLane/18(line03_C3)
  line03_C2/1 -> ObjToCenterLine_dyc_LeftLane/17(line03_C2)
  line03_C1/1 -> ObjToCenterLine_dyc_LeftLane/16(line03_C1)
  line03_C0/1 -> ObjToCenterLine_dyc_LeftLane/15(line03_C0)
  line02_dDisEnd/1 -> ObjToCenterLine_dyc_LeftLane/14(line02_dDisEnd)
  line02_dDisStart/1 -> ObjToCenterLine_dyc_LeftLane/13(line02_dDisStart)
  line02_C3/1 -> ObjToCenterLine_dyc_LeftLane/12(line02_C3)
  line02_C2/1 -> ObjToCenterLine_dyc_LeftLane/11(line02_C2)
  line02_C1/1 -> ObjToCenterLine_dyc_LeftLane/10(line02_C1)
  line02_C0/1 -> ObjToCenterLine_dyc_LeftLane/9(line02_C0)
  line01_dDisEnd/1 -> ObjToCenterLine_dyc_LeftLane/8(line01_dDisEnd)
  line01_dDisStart/1 -> ObjToCenterLine_dyc_LeftLane/7(line01_dDisStart)
  line01_C3/1 -> ObjToCenterLine_dyc_LeftLane/6(line01_C3)
  line01_C2/1 -> ObjToCenterLine_dyc_LeftLane/5(line01_C2)
  line01_C1/1 -> ObjToCenterLine_dyc_LeftLane/4(line01_C1)
  line01_C0/1 -> ObjToCenterLine_dyc_LeftLane/3(line01_C0)
  Object_DX/1 -> ObjToCenterLine_dyc_LeftLane/2(Object_DX)
  Object_DY/1 -> ObjToCenterLine_dyc_LeftLane/1(Object_DY)

== system PubIfDecisionTOS_MDL/TOS_20201112/TOS_2012080320/PIL_1029/BoundaryCalculat/ObjectToCenterLine_dyc/LeftLane/PIL_ObjectToCenterLine_dy_Filt ==
  note: fun: 目标到本车道中心线距离滤波
  TOS_OFMObjValid_Flag : Inport
  Object_ID : Inport  Port=2  OutDataTypeStr=uint8
  Object_Age : Inport  Port=3
  ObjectToCenterLine_dy : Inport  Port=4
  PIL_ObjectToCenterLine_dy : Subsystem
  Unit Delay : UnitDelay  InitialCondition=zeros(80,1)  SampleTime=-1  HasFrameUpgradeWarning=on
      settings: AttributesFormatString=initVal = zeros(80,1)
  Unit Delay1 : UnitDelay  InitialCondition=ones(80,1)*255  SampleTime=-1  HasFrameUpgradeWarning=on
      settings: AttributesFormatString=initVal = ones(80,1)*255
  PIL_ObjectToCenterLine_dy_Filt : Outport  OutDataTypeStr=single
  wires:
  TOS_OFMObjValid_Flag/1 -> PIL_ObjectToCenterLine_dy/4(TOS_OFMObjValid_Flag)
  Object_Age/1 -> PIL_ObjectToCenterLine_dy/6(Object_Age)
  ObjectToCenterLine_dy/1 -> PIL_ObjectToCenterLine_dy/3(ObjectToCenterLine_dy)
  PIL_ObjectToCenterLine_dy/2(ObjectToCenterLine_dy_Filt) -> PIL_ObjectToCenterLine_dy_Filt/1, Unit Delay1/1
  Unit Delay1/1 -> PIL_ObjectToCenterLine_dy/2(ObjectToCenterLine_dy_Filt_K1)
  Object_ID/1 -> PIL_ObjectToCenterLine_dy/5(Object_ID)
  PIL_ObjectToCenterLine_dy/1(Obj_ID) -> Unit Delay/1
  Unit Delay/1 -> PIL_ObjectToCenterLine_dy/1(ObjectID_Filt_K1)

== system PubIfDecisionTOS_MDL/TOS_20201112/TOS_2012080320/PIL_1029/BoundaryCalculat/ObjectToCenterLine_dyc/RightLane/PIL_ObjectToCenterLine_dy_Filt ==
  note: fun: 目标到本车道中心线距离滤波
  TOS_OFMObjValid_Flag : Inport
  Object_ID : Inport  Port=2  OutDataTypeStr=uint8
  Object_Age : Inport  Port=3
  ObjectToCenterLine_dy : Inport  Port=4
  PIL_ObjectToCenterLine_dy : Subsystem
  Unit Delay : UnitDelay  InitialCondition=zeros(80,1)  SampleTime=-1  HasFrameUpgradeWarning=on
      settings: AttributesFormatString=initVal = zeros(80,1)
  Unit Delay1 : UnitDelay  InitialCondition=ones(80,1)*255  SampleTime=-1  HasFrameUpgradeWarning=on
      settings: AttributesFormatString=initVal = ones(80,1)*255
  PIL_ObjectToCenterLine_dy_Filt : Outport  OutDataTypeStr=single
  wires:
  TOS_OFMObjValid_Flag/1 -> PIL_ObjectToCenterLine_dy/4(TOS_OFMObjValid_Flag)
  Object_Age/1 -> PIL_ObjectToCenterLine_dy/6(Object_Age)
  ObjectToCenterLine_dy/1 -> PIL_ObjectToCenterLine_dy/3(ObjectToCenterLine_dy)
  PIL_ObjectToCenterLine_dy/2(ObjectToCenterLine_dy_Filt) -> PIL_ObjectToCenterLine_dy_Filt/1, Unit Delay1/1
  Unit Delay1/1 -> PIL_ObjectToCenterLine_dy/2(ObjectToCenterLine_dy_Filt_K1)
  Object_ID/1 -> PIL_ObjectToCenterLine_dy/5(Object_ID)
  PIL_ObjectToCenterLine_dy/1(Obj_ID) -> Unit Delay/1
  Unit Delay/1 -> PIL_ObjectToCenterLine_dy/1(ObjectID_Filt_K1)

== system PubIfDecisionTOS_MDL/TOS_20201112/TOS_2012080320/PIL_1029/BoundaryCalculat/ObjectToCenterLine_dyc/RightLane/RightCenterLine_dyc ==
  TOS_OFMObjValid_Flag : Inport  Partition=on  PartitionDimension=1  PartitionWidth=1  PartitionOffset=0
  Object_DY : Inport  Port=2  Partition=on  PartitionDimension=1  PartitionWidth=1  PartitionOffset=0
  Object_DX : Inport  Port=3  Partition=on  PartitionDimension=1  PartitionWidth=1  PartitionOffset=0
  line01_C0 : Inport  Port=4
  line01_C1 : Inport  Port=5
  line01_C2 : Inport  Port=6
  line01_C3 : Inport  Port=7
  line01_dDisStart : Inport  Port=8
  line01_dDisEnd : Inport  Port=9
  line02_C0 : Inport  Port=10
  line02_C1 : Inport  Port=11
  line02_C2 : Inport  Port=12
  line02_C3 : Inport  Port=13
  line02_dDisStart : Inport  Port=14
  line02_dDisEnd : Inport  Port=15
  line03_C0 : Inport  Port=16
  line03_C1 : Inport  Port=17
  line03_C2 : Inport  Port=18
  line03_C3 : Inport  Port=19
  line03_dDisStart : Inport  Port=20
  line03_dDisEnd : Inport  Port=21
  line04_C0 : Inport  Port=22
  line04_C1 : Inport  Port=23
  line04_C2 : Inport  Port=24
  line04_C3 : Inport  Port=25
  line04_dDisStart : Inport  Port=26
  line04_dDisEnd : Inport  Port=27
  line05_C0 : Inport  Port=28
  line05_C1 : Inport  Port=29
  line05_C2 : Inport  Port=30
  line05_C3 : Inport  Port=31
  line05_dDisStart : Inport  Port=32
  line05_dDisEnd : Inport  Port=33
  line06_C0 : Inport  Port=34
  line06_C1 : Inport  Port=35
  line06_C2 : Inport  Port=36
  line06_C3 : Inport  Port=37
  line06_dDisStart : Inport  Port=38
  line06_dDisEnd : Inport  Port=39
  Compare To Constant : simulink/Logic and Bit Operations/Compare To Constant  relop===  const=C_TOS_OFMObjIDInvilad_Val  OutDataTypeStr=boolean
      settings: AttributesFormatString=C_TOS_OFMObjIDInvilad_Val = 0
  For Each : ForEach  DisableCoverage=on
  If : If  IfExpression=u1 ~= 0
  Merge : Merge
  ObjToCenterLine_dyc_RightLane : Subsystem
  ObjToCenterLine_dyc_RightLaneDefault : Subsystem  TreatAsAtomicUnit=on
  ObjectToCenterLine_dyc_RightLane : Outport  ConcatenationDimension=1
  wires:
  Object_DY/1 -> ObjToCenterLine_dyc_RightLane/1(Object_DY)
  Object_DX/1 -> ObjToCenterLine_dyc_RightLane/2(Object_DX)
  line01_C0/1 -> ObjToCenterLine_dyc_RightLane/3(line01_C0)
  line01_C1/1 -> ObjToCenterLine_dyc_RightLane/4(line01_C1)
  line01_C2/1 -> ObjToCenterLine_dyc_RightLane/5(line01_C2)
  line01_C3/1 -> ObjToCenterLine_dyc_RightLane/6(line01_C3)
  line01_dDisStart/1 -> ObjToCenterLine_dyc_RightLane/7(line01_dDisStart)
  line01_dDisEnd/1 -> ObjToCenterLine_dyc_RightLane/8(line01_dDisEnd)
  line02_C0/1 -> ObjToCenterLine_dyc_RightLane/9(line02_C0)
  line02_C1/1 -> ObjToCenterLine_dyc_RightLane/10(line02_C1)
  line02_C2/1 -> ObjToCenterLine_dyc_RightLane/11(line02_C2)
  line02_C3/1 -> ObjToCenterLine_dyc_RightLane/12(line02_C3)
  line02_dDisStart/1 -> ObjToCenterLine_dyc_RightLane/13(line02_dDisStart)
  line02_dDisEnd/1 -> ObjToCenterLine_dyc_RightLane/14(line02_dDisEnd)
  line03_C0/1 -> ObjToCenterLine_dyc_RightLane/15(line03_C0)
  line03_C1/1 -> ObjToCenterLine_dyc_RightLane/16(line03_C1)
  line03_C2/1 -> ObjToCenterLine_dyc_RightLane/17(line03_C2)
  line03_C3/1 -> ObjToCenterLine_dyc_RightLane/18(line03_C3)
  line03_dDisStart/1 -> ObjToCenterLine_dyc_RightLane/19(line03_dDisStart)
  line03_dDisEnd/1 -> ObjToCenterLine_dyc_RightLane/20(line03_dDisEnd)
  line04_C0/1 -> ObjToCenterLine_dyc_RightLane/21(line04_C0)
  line04_C1/1 -> ObjToCenterLine_dyc_RightLane/22(line04_C1)
  line04_C2/1 -> ObjToCenterLine_dyc_RightLane/23(line04_C2)
  line04_C3/1 -> ObjToCenterLine_dyc_RightLane/24(line04_C3)
  line04_dDisStart/1 -> ObjToCenterLine_dyc_RightLane/25(line04_dDisStart)
  line04_dDisEnd/1 -> ObjToCenterLine_dyc_RightLane/26(line04_dDisEnd)
  line05_C0/1 -> ObjToCenterLine_dyc_RightLane/27(line05_C0)
  line05_C1/1 -> ObjToCenterLine_dyc_RightLane/28(line05_C1)
  line05_C2/1 -> ObjToCenterLine_dyc_RightLane/29(line05_C2)
  line05_C3/1 -> ObjToCenterLine_dyc_RightLane/30(line05_C3)
  line05_dDisStart/1 -> ObjToCenterLine_dyc_RightLane/31(line05_dDisStart)
  line05_dDisEnd/1 -> ObjToCenterLine_dyc_RightLane/32(line05_dDisEnd)
  line06_C0/1 -> ObjToCenterLine_dyc_RightLane/33(line06_C0)
  line06_C1/1 -> ObjToCenterLine_dyc_RightLane/34(line06_C1)
  line06_C2/1 -> ObjToCenterLine_dyc_RightLane/35(line06_C2)
  line06_C3/1 -> ObjToCenterLine_dyc_RightLane/36(line06_C3)
  line06_dDisStart/1 -> ObjToCenterLine_dyc_RightLane/37(line06_dDisStart)
  line06_dDisEnd/1 -> ObjToCenterLine_dyc_RightLane/38(line06_dDisEnd)
  ObjToCenterLine_dyc_RightLane/1(ObjectToCenterLine_dyc_RightLane) -> Merge/2
  If/1 -> ObjToCenterLine_dyc_RightLaneDefault/Action
  Compare To Constant/1 -> If/1
  If/2 -> ObjToCenterLine_dyc_RightLane/Action
  TOS_OFMObjValid_Flag/1 -> Compare To Constant/1
  Merge/1 -> ObjectToCenterLine_dyc_RightLane/1
  ObjToCenterLine_dyc_RightLaneDefault/1(ObjectToCenterLine_dyc_LeftLane) -> Merge/1
